simulink model "LyapunovTesteSigns"  (R2016a)
settings: Solver=ode23t  StartTime=0.0  StopTime=10  FixedStep=t_PWM/10  MaxStep=2e-6  RelTol=2e-4
values from neighbouring files (symbols this model uses):
  C1 = t_PWM * (N*Impp)*0.1/ (8 * (N*Vmpp)*0.0001)    [SolarPanelModel.m]
  C2 = (N*Vo) * t_PWM/ (Load * (N*Vo)*0.001)    [SolarPanelModel.m]
  delta_Il = (N*Impp)*0.1/ 2    [SolarPanelModel.m]
  G = 1000    [SolarPanelModel.m]
  Gr = 1000    [SolarPanelModel.m]
  Isc = G/ Gr * (Iscr + miu_Isc*(Tc - Tr))    (= 9.318625)    [SolarPanelModel.m]
  Iscr = 9.19    [SolarPanelModel.m]
  K = 1.38 * 10^(-23)    (= 1.38e-23)    [SolarPanelModel.m]
  k_l = k_v/10    (= 2)    [SolarPanelModel.m]
  L_inductor = (N*Vo) * t_PWM/ (4 * (N*Impp)*0.01)    [SolarPanelModel.m]
  m = sol(1)    [SolarPanelModel.m]
  miu_Isc = 0.0049    [SolarPanelModel.m]
  miu_Voc = -0.1184    [SolarPanelModel.m]
  N = 3    [SolarPanelModel.m]
  NOCT = 45    [SolarPanelModel.m]
  q = 1.6 * 10^(-19)    (= 1.6e-19)    [SolarPanelModel.m]
  Rs = sol(3)    [SolarPanelModel.m]
  Rsh = sol(2)    [SolarPanelModel.m]
  T = 273.15    [SolarPanelModel.m]
  t_PWM = 20e-6    (= 2e-05)    [SolarPanelModel.m]
  ta = 20    [SolarPanelModel.m]
  Tr = T + 25    (= 298.15)    [SolarPanelModel.m]
  Vmpp = V(ind)    [SolarPanelModel.m]
  Voc = Vocr + miu_Voc*(Tc - Tr) + m*Vt*log(G/Gr)    [SolarPanelModel.m]
  Vocr = 38.2    [SolarPanelModel.m]
undefined symbols (not defined in the file or in its folder): ki_ig, kv_ig
libraries: powerlib x20, powerlib_extras x9
settings Model: Creator=frede  LastModifiedBy=frede
settings DataIOCC: LimitDataPoints=on  SaveFormat=Array
settings HardwareCC: ProdBitPerPointer=32  ProdLargestAtomicFloat=None  ProdIntDivRoundTo=Undefined  ProdEndianess=Unspecified  ProdWordSize=32  ProdHWDeviceType=32-bit Generic
settings ModelReferenceCC: PropagateSignalLabelsOutOfModel=off
settings ConfigComp: CovModelRefEnable=Off

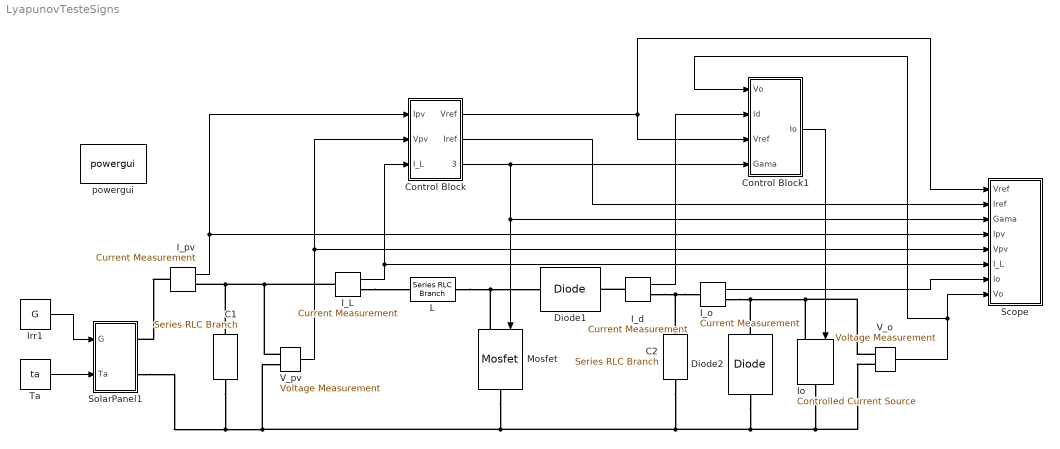
== system LyapunovTesteSigns ==
  C1 : powerlib/Elements/Series RLC Branch  LConnTagsString=__new0  RConnTagsString=__new0  BranchType=C  Resistance=Rs  Inductance=1e-3  SetiL0=off  InitialCurrent=0  Capacitance=C1  Setx0=off  InitialVoltage=0  Measurements=None
  C2 : powerlib/Elements/Series RLC Branch  LConnTagsString=__new0  RConnTagsString=__new0  BranchType=C  Resistance=Rs  Inductance=1e-3  SetiL0=off  InitialCurrent=0  Capacitance=C2  Setx0=off  InitialVoltage=0  Measurements=None
  Control Block : Subsystem
  Control Block1 : Subsystem
  Diode1 : powerlib/Power Electronics/Diode  Ron=0.001  Lon=0  Vf=0.001  IC=0  UseSnubber=off  Rs=500  Cs=2e-9  Measurements=off
  Diode2 : powerlib/Power Electronics/Diode  Ron=0.001  Lon=0  Vf=0.001  IC=0  UseSnubber=off  Rs=500  Cs=2e-9  Measurements=off
  I_L : powerlib/Measurements/Current Measurement  PhasorSimulation=off  OutputType=Complex  PSBequivalent=0
  I_d : powerlib/Measurements/Current Measurement  PhasorSimulation=off  OutputType=Complex  PSBequivalent=0
  I_o : powerlib/Measurements/Current Measurement  PhasorSimulation=off  OutputType=Complex  PSBequivalent=0
  I_pv : powerlib/Measurements/Current Measurement  PhasorSimulation=off  OutputType=Complex  PSBequivalent=0
  Io : powerlib/Electrical Sources/Controlled Current Source  Initialize=on  Source_Type=AC  Amplitude=0  Phase=0  Frequency=0  Measurements=None
  Irr1 : Constant  Value=G
  L : powerlib/Elements/Series RLC Branch  LConnTagsString=__new0  RConnTagsString=__new0  BranchType=L  Resistance=Rs  Inductance=L_inductor  SetiL0=off  InitialCurrent=0  Capacitance=1e-6  Setx0=off  InitialVoltage=0  Measurements=None
  Mosfet : powerlib/Power Electronics/Mosfet  Ron=0.001  Lon=0  Rd=0.001  Vfd=0  IC=0  Rs=1e3  Cs=1e-7  Measurements=off
  Scope : Subsystem
  SolarPanel1 : Subsystem
  Ta : Constant  Value=ta
  V_o : powerlib/Measurements/Voltage Measurement  PhasorSimulation=off  OutputType=Complex  PSBequivalent=0
  V_pv : powerlib/Measurements/Voltage Measurement  PhasorSimulation=off  OutputType=Complex  PSBequivalent=0
  powergui : powerlib/powergui  Priority=1  SimulationMode=Discrete  SolverType=Tustin/Backward Euler (TBE)  SampleTime=t_PWM/10  frequency=60  SPID=off  DisableSnubberDevices=off  DisableRonSwitches=off  DisableVfSwitches=off  SwTol=0  DisplayEquations=off  Interpol=off  ExternalGateDelay=off  methode=off  Ts=10  FunctionMessages=off  echomessages=off  HookPort=off  EnableUseOfTLC=off  x0status=blocks  frequencyindice=0  Pbase=100e6  ErrMax=1e-4  Iterations=50  UnitsV=kV  UnitsW=MW  buscounter=0  RestoreLinks=warning  ResistiveCurrentMeasurement=off  Frange=[0:2:500]  Ylog=off  Xlog=on  ShowGrid=off  save=off  variable=ZData  structure=0  ZoomFFT=off  StartTime=0.0  cycles=1  DisplayStyle=1  fundamental=60  FreqAxis=off  MaxFrequency=1000  frequencyindicesteady=1  RmsSteady=1  display=off
  wires:
  I_L/1 -> Control Block/3(I_L), Scope/6(I_L)
  V_o/1 -> Control Block1/1(Vo), Scope/8(Vo)
  Ta/1 -> SolarPanel1/2(Ta)
  Irr1/1 -> SolarPanel1/1(G)
  Control Block/3(Gama) -> Control Block1/4(Gama), Mosfet/1, Scope/3(Gama)
  I_pv/1 -> Control Block/1(Ipv), Scope/4(Ipv)
  V_pv/1 -> Scope/5(Vpv), Control Block/2(Vpv)
  I_o/1 -> Scope/7(Io)
  Control Block1/1(Io) -> Io/1
  I_d/1 -> Control Block1/2(Id)
  Control Block/1(Vref) -> Control Block1/3(Vref), Scope/1(Vref)
  Control Block/2(Iref) -> Scope/2(Iref)
  connections:
  V_pv/LConn1 -- I_L/LConn1 -- C1/LConn1 -- I_pv/RConn1
  Io/RConn1 -- V_o/LConn2 -- Diode2/LConn1 -- C1/RConn1 -- SolarPanel1/RConn2 -- V_pv/LConn2 -- Mosfet/RConn1 -- C2/RConn1
  L/RConn1 -- Diode1/LConn1 -- Mosfet/LConn1
  I_L/RConn1 -- L/LConn1
  I_pv/LConn1 -- SolarPanel1/RConn1
  Io/LConn1 -- V_o/LConn1 -- Diode2/RConn1 -- I_o/RConn1
  I_o/LConn1 -- I_d/RConn1 -- C2/LConn1
  I_d/LConn1 -- Diode1/RConn1

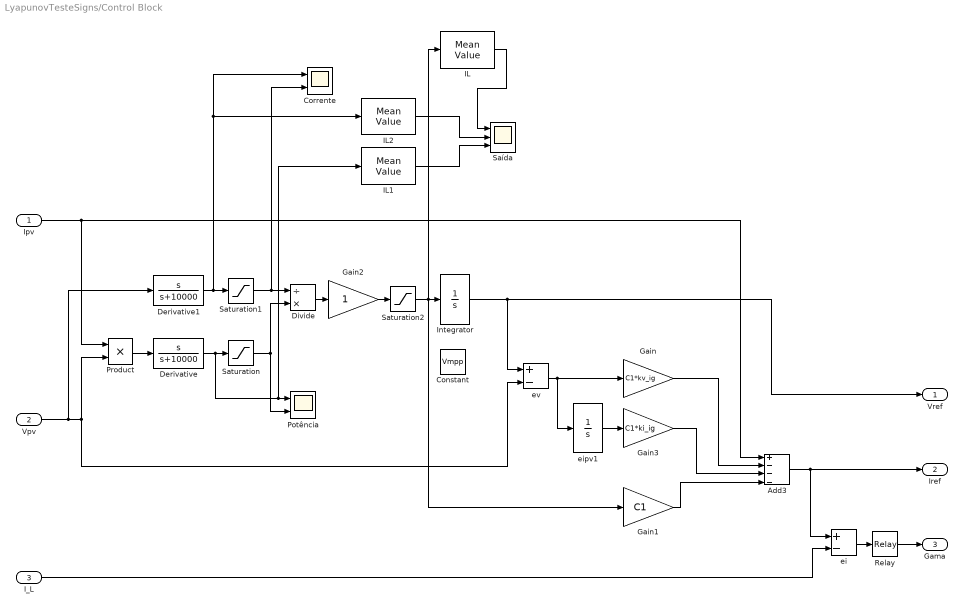
== system LyapunovTesteSigns/Control Block ==
  Ipv : Inport
  Vpv : Inport  Port=2
  I_L : Inport  Port=3
  Add3 : Sum  Inputs=+---
  Constant : Constant  Value=Vmpp
  Corrente : Scope  NumInputPorts=2
  Derivative : TransferFcn  Numerator=[1 0]  Denominator=[1 10000]
  Derivative1 : TransferFcn  Numerator=[1 0]  Denominator=[1 10000]
  Divide : Product  Inputs=/*
  Gain : Gain  Gain=C1*kv_ig
  Gain1 : Gain  Gain=C1
  Gain2 : Gain
  Gain3 : Gain  Gain=C1*ki_ig
  IL : powerlib_extras/Measurements/Mean Value  Period=1/100
  IL1 : powerlib_extras/Measurements/Mean Value  Period=1/10
  IL2 : powerlib_extras/Measurements/Mean Value  Period=1/10
  Integrator : Integrator  InitialCondition=Voc*0.5  LimitOutput=on  UpperSaturationLimit=Voc  LowerSaturationLimit=0
  Potência : Scope  NumInputPorts=2
  Product : Product  Inputs=**
  Relay : Relay  OnSwitchValue=delta_Il*0.1  OffSwitchValue=-delta_Il*0.1
  Saturation : Saturate  UpperLimit=1  LowerLimit=-1
  Saturation1 : Saturate  UpperLimit=1  LowerLimit=-1
  Saturation2 : Saturate  UpperLimit=5  LowerLimit=-5
  Saída : Scope  NumInputPorts=3
  ei : Sum  Inputs=+-
  eipv1 : Integrator  UpperSaturationLimit=Voc*N  LowerSaturationLimit=0
  ev : Sum  Inputs=+-
  Vref : Outport
  Iref : Outport  Port=2
  Gama : Outport  Port=3
  wires:
  ev/1 -> eipv1/1, Gain/1
  Gain/1 -> Add3/2
  Gain1/1 -> Add3/4
  Divide/1 -> Gain2/1
  Ipv/1 -> Add3/1, Product/1
  Vpv/1 -> Product/2, ev/2, Derivative1/1
  Integrator/1 -> ev/1, Vref/1
  eipv1/1 -> Gain3/1
  Gain3/1 -> Add3/3
  Add3/1 -> Iref/1, ei/1
  I_L/1 -> ei/2
  ei/1 -> Relay/1
  Relay/1 -> Gama/1
  IL/1 -> Saída/1
  Product/1 -> Derivative/1
  Derivative/1 -> Saturation/1, IL1/1, Potência/1
  Saturation/1 -> Potência/2, Divide/2
  Derivative1/1 -> IL2/1, Corrente/1, Saturation1/1
  Saturation1/1 -> Corrente/2, Divide/1
  Gain2/1 -> Saturation2/1
  Saturation2/1 -> Gain1/1, IL/1, Integrator/1
  IL1/1 -> Saída/3
  IL2/1 -> Saída/2

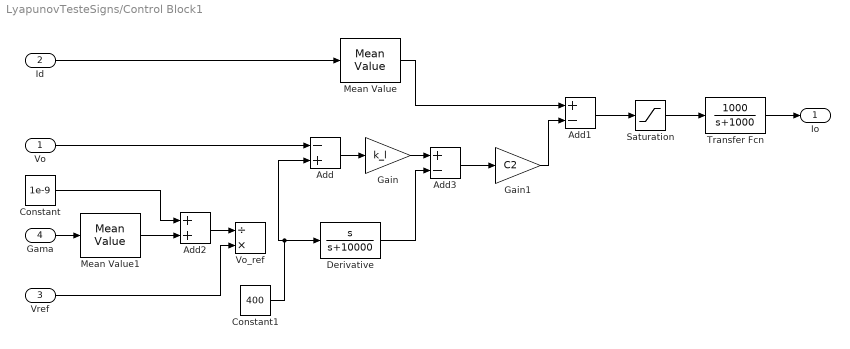
== system LyapunovTesteSigns/Control Block1 ==
  Vo : Inport
  Id : Inport  Port=2
  Vref : Inport  Port=3
  Gama : Inport  Port=4
  Add : Sum  Inputs=-+
  Add1 : Sum  Inputs=+-
  Add2 : Sum
  Add3 : Sum  Inputs=+-
  Constant : Constant  Value=1e-9
  Constant1 : Constant  Value=400
  Derivative : TransferFcn  Numerator=[1 0]  Denominator=[1 10000]
  Gain : Gain  Gain=k_l
  Gain1 : Gain  Gain=C2
  Mean Value : powerlib_extras/Measurements/Mean Value  Period=1/100
  Mean Value1 : powerlib_extras/Measurements/Mean Value  Period=1/100
  Saturation : Saturate  UpperLimit=Isc  LowerLimit=0
  Transfer Fcn : TransferFcn  Numerator=[1000]  Denominator=[1 1000]
  Vo_ref : Product  Inputs=/*
  Io : Outport
  wires:
  Vo/1 -> Add/1
  Add/1 -> Gain/1
  Id/1 -> Mean Value/1
  Add1/1 -> Saturation/1
  Mean Value/1 -> Add1/1
  Gama/1 -> Mean Value1/1
  Vref/1 -> Vo_ref/2
  Constant1/1 -> Add/2, Derivative/1
  Add2/1 -> Vo_ref/1
  Mean Value1/1 -> Add2/2
  Gain/1 -> Add3/1
  Derivative/1 -> Add3/2
  Saturation/1 -> Transfer Fcn/1
  Transfer Fcn/1 -> Io/1
  Constant/1 -> Add2/1
  Add3/1 -> Gain1/1
  Gain1/1 -> Add1/2

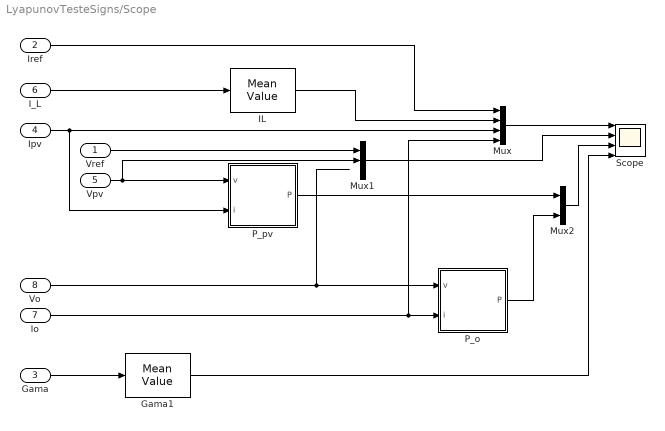
== system LyapunovTesteSigns/Scope ==
  Vref : Inport
  Iref : Inport  Port=2
  Gama : Inport  Port=3
  Ipv : Inport  Port=4
  Vpv : Inport  Port=5
  I_L : Inport  Port=6
  Io : Inport  Port=7
  Vo : Inport  Port=8
  Gama1 : powerlib_extras/Measurements/Mean Value  Period=1/100
  IL : powerlib_extras/Measurements/Mean Value  Period=1/100
  Mux : Mux
  Mux1 : Mux  Inputs=3
  Mux2 : Mux  Inputs=2
  P_o : Subsystem
  P_pv : Subsystem
  Scope : Scope  NumInputPorts=4
  wires:
  Mux/1 -> Scope/1
  Mux2/1 -> Scope/3
  P_pv/1(P) -> Mux2/1
  Io/1 -> Mux/4, P_o/2(i)
  Mux1/1 -> Scope/2
  Vo/1 -> P_o/1(v)
  Ipv/1 -> Mux/3, P_pv/2(i)
  Vpv/1 -> Mux1/2, P_pv/1(v)
  Vref/1 -> Mux1/1
  P_o/1(P) -> Mux2/2
  I_L/1 -> IL/1
  IL/1 -> Mux/2
  Iref/1 -> Mux/1
  Gama/1 -> Gama1/1
  Gama1/1 -> Scope/4

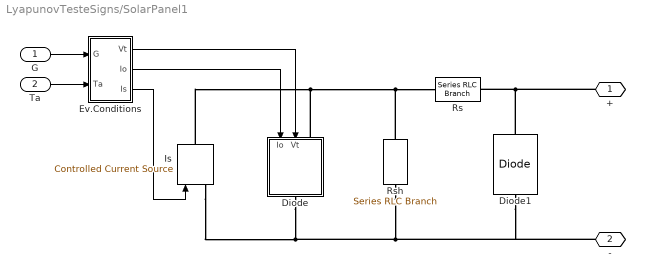
== system LyapunovTesteSigns/SolarPanel1 ==
  G : Inport
  Ta : Inport  Port=2
  Diode : Subsystem  AncestorBlock=re_lib/Solar/PV Array/Diode Rsh
      mask Display:
      | plot(-75,-50,100,150, [-15 -15 43 -15 -15 -75],[50 8 50 92 50 50], ...
      |     [43 43],[8 94],[100 43], [50 50])
  Diode1 : powerlib/Power Electronics/Diode  Ron=0.001  Lon=0  Vf=0  IC=0  UseSnubber=off  Rs=500  Cs=250e-9  Measurements=off
  Ev.Conditions : Subsystem
  Is : powerlib/Electrical Sources/Controlled Current Source  Initialize=on  Source_Type=DC  Amplitude=0  Phase=0  Frequency=0  Measurements=None
  Rs : powerlib/Elements/Series RLC Branch  LConnTagsString=__new0  RConnTagsString=__new0  BranchType=R  Resistance=Rs  Inductance=1e-3  SetiL0=off  InitialCurrent=0  Capacitance=1e-6  Setx0=off  InitialVoltage=0  Measurements=None
  Rsh : powerlib/Elements/Series RLC Branch  LConnTagsString=__new0  RConnTagsString=__new0  BranchType=R  Resistance=Rsh  Inductance=1e-3  SetiL0=off  InitialCurrent=0  Capacitance=1e-6  Setx0=off  InitialVoltage=0  Measurements=None
  + : PMIOPort  Port=1  Side=Right
  - : PMIOPort  Port=2  Side=Right
  wires:
  G/1 -> Ev.Conditions/1(G)
  Ta/1 -> Ev.Conditions/2(Ta)
  Ev.Conditions/2(Io) -> Diode/1(Io)
  Ev.Conditions/1(Vt) -> Diode/2(Vt)
  Ev.Conditions/3(Is) -> Is/1
  connections:
  Is/RConn1 -- Diode/LConn1 -- Rsh/LConn1 -- Rs/LConn1
  Rsh/RConn1 -- -/RConn1 -- Diode1/LConn1 -- Is/LConn1 -- Diode/RConn1
  Diode1/RConn1 -- Rs/RConn1 -- +/RConn1

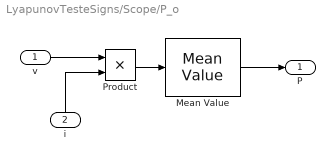
== system LyapunovTesteSigns/Scope/P_o ==
  v : Inport
  i : Inport  Port=2
  Mean Value : powerlib_extras/Measurements/Mean Value  Period=1/100
  Product : Product
  P : Outport
  wires:
  Mean Value/1 -> P/1
  Product/1 -> Mean Value/1
  v/1 -> Product/1
  i/1 -> Product/2

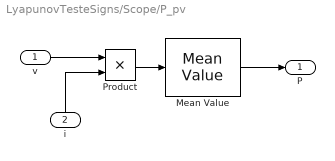
== system LyapunovTesteSigns/Scope/P_pv ==
  v : Inport
  i : Inport  Port=2
  Mean Value : powerlib_extras/Measurements/Mean Value  Period=1/100
  Product : Product
  P : Outport
  wires:
  Mean Value/1 -> P/1
  Product/1 -> Mean Value/1
  v/1 -> Product/1
  i/1 -> Product/2

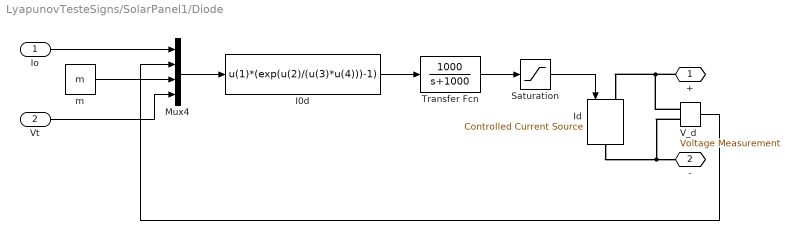
== system LyapunovTesteSigns/SolarPanel1/Diode ==
  Io : Inport
  Vt : Inport  Port=2
  I0d : Fcn  Expr=u(1)*(exp(u(2)/(u(3)*u(4)))-1)
  Id : powerlib/Electrical Sources/Controlled Current Source  Initialize=on  Source_Type=DC  Amplitude=0  Phase=0  Frequency=0  Measurements=None
  Mux4 : Mux
  Saturation : Saturate  UpperLimit=Isc  LowerLimit=0
  Transfer Fcn : TransferFcn  Numerator=[1000]  Denominator=[1 1000]
  V_d : powerlib/Measurements/Voltage Measurement  PhasorSimulation=off  OutputType=Complex  PSBequivalent=0
  m : Constant  Value=m
  + : PMIOPort  Port=1  Side=Left
  - : PMIOPort  Port=2  Side=Right
  wires:
  Mux4/1 -> I0d/1
  Io/1 -> Mux4/1
  V_d/1 -> Mux4/2
  m/1 -> Mux4/3
  Vt/1 -> Mux4/4
  I0d/1 -> Transfer Fcn/1
  Transfer Fcn/1 -> Saturation/1
  Saturation/1 -> Id/1
  connections:
  Id/RConn1 -- V_d/LConn2 -- -/RConn1
  +/RConn1 -- V_d/LConn1 -- Id/LConn1

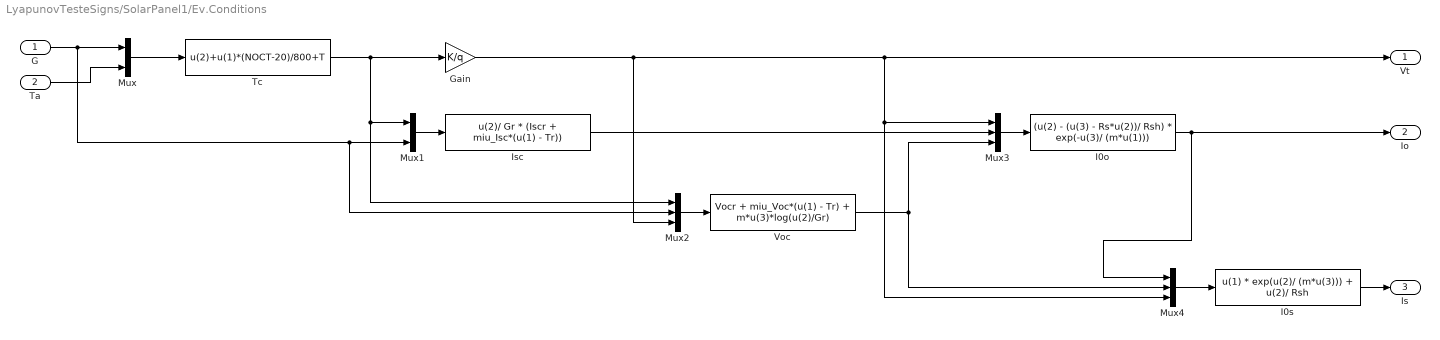
== system LyapunovTesteSigns/SolarPanel1/Ev.Conditions ==
  G : Inport
  Ta : Inport  Port=2
  Gain : Gain  Gain=K/q
  I0o : Fcn  Expr=(u(2) - (u(3) - Rs*u(2))/ Rsh) * exp(-u(3)/ (m*u(1)))
  I0s : Fcn  Expr=u(1) * exp(u(2)/ (m*u(3))) + u(2)/ Rsh
  Isc : Fcn  Expr=u(2)/ Gr * (Iscr + miu_Isc*(u(1) - Tr))
  Mux : Mux  Inputs=2
  Mux1 : Mux  Inputs=2
  Mux2 : Mux  Inputs=3
  Mux3 : Mux  Inputs=3
  Mux4 : Mux  Inputs=3
  Tc : Fcn  Expr=u(2)+u(1)*(NOCT-20)/800+T
  Voc : Fcn  Expr=Vocr + miu_Voc*(u(1) - Tr) + m*u(3)*log(u(2)/Gr)
  Vt : Outport
  Io : Outport  Port=2
  Is : Outport  Port=3
  wires:
  Mux1/1 -> Isc/1
  Gain/1 -> Mux2/3, Vt/1, Mux4/3, Mux3/1
  Mux/1 -> Tc/1
  I0s/1 -> Is/1
  Ta/1 -> Mux/2
  G/1 -> Mux/1, Mux2/2, Mux1/2
  Tc/1 -> Mux2/1, Mux1/1, Gain/1
  I0o/1 -> Mux4/1, Io/1
  Mux2/1 -> Voc/1
  Mux3/1 -> I0o/1
  Isc/1 -> Mux3/2
  Voc/1 -> Mux3/3, Mux4/2
  Mux4/1 -> I0s/1
